simulink model "mpc_test_dist_rej"  (R2024b)
settings: Solver=FixedStepDiscrete  StartTime=0.0  StopTime=10  FixedStep=0.01  RelTol=1e-3  EnableMultiTasking=on
values from neighbouring files (symbols this model uses):
  A_aug = [str_discr_sys.A,str_discr_sys.B ... (first row only)    [MPC_controller.m]    (also in MPC_controller_withint_testing.m)
  B_aug = [str_discr_sys.B;0]    [MPC_controller.m]    (also in MPC_controller_withint_testing.m)
  C_aug = [str_discr_sys.C, zeros(2,1)]    [MPC_controller.m]    (also in MPC_controller_withint_testing.m)
  D_aug = str_discr_sys.D    [MPC_controller.m]    (also in MPC_controller_withint_testing.m)
  h = log(abs(sec(theta)+tan(theta))-C1*alpha)    [Design_of_nonlinear_controller.m]    (also in MPC_controller.m = 0.01; MPC_controller_withint_testing.m = 0.01)
undefined symbols (not defined in the file or in its folder): Discrete, Time
libraries: ctrlSharedLib x1, cstblocks x1
settings Model: Creator=rbabuska  LastModifiedBy=Wesley
settings SolverCC: AlgebraicLoopSolver=TrustRegion
settings DataIOCC: LimitDataPoints=on  SaveFormat=Array  SignalLoggingSaveFormat=ModelDataLogs  ReturnWorkspaceOutputs=off
settings OptimizationCC: ExpressionDepthLimit=2147483647  LifeSpan=inf
settings DebuggingCC: UnderspecifiedInitializationDetection=Classic  MergeDetectMultiDrivingBlocksExec=none  FcnCallInpInsideContextMsg=warning  UnconnectedInputMsg=warning  UnconnectedOutputMsg=warning  UnconnectedLineMsg=warning  StateNameClashWarn=warning  SFUnexpectedBacktrackingDiag=warning  SFNoUnconditionalDefaultTransitionDiag=warning  SFExecutionAtInitializationDiag=none  ArithmeticOperatorsInVariantConditions=warning
settings HardwareCC: ProdBitPerPointer=32  ProdBitPerSizeT=32  ProdBitPerPtrDiffT=32  ProdLargestAtomicFloat=None  ProdIntDivRoundTo=Undefined  ProdEndianess=Unspecified  ProdWordSize=32  ProdHWDeviceType=32-bit Generic
settings ModelReferenceCC: EnableRefExpFcnMdlSchedulingChecks=on  PropagateSignalLabelsOutOfModel=off
settings SFSimCC: SimUseLocalCustomCode=off  CustomCodeUndefinedFunction=UseInterfaceOnly
settings RTWCC: RTWUseLocalCustomCode=off  GPUComputeCapability=3.5  DLArmComputeVersion=19.05
settings CodeAppCC: StateflowObjectComments=on
settings GRTTargetCC: TargetLangStandard=C89/C90 (ANSI)  CombineOutputUpdateFcns=off  GRTInterface=on
settings ConfigComp: CovMetricSettings=dw  CovSaveCumulativeToWorkspaceVar=on  CovSaveSingleToWorkspaceVar=on  CovExternalEMLEnable=off  CovSFcnEnable=off

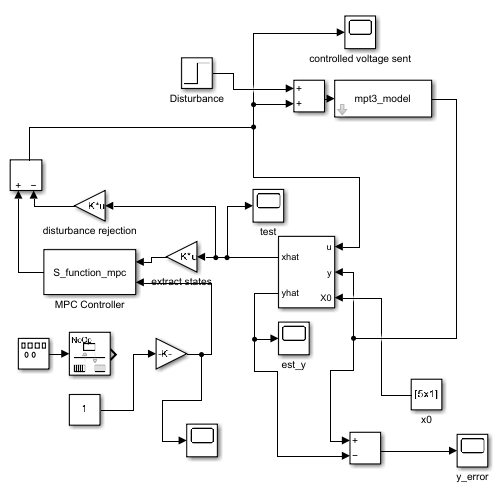
[thumbnail: Simulink's stored preview of the top-level diagram]
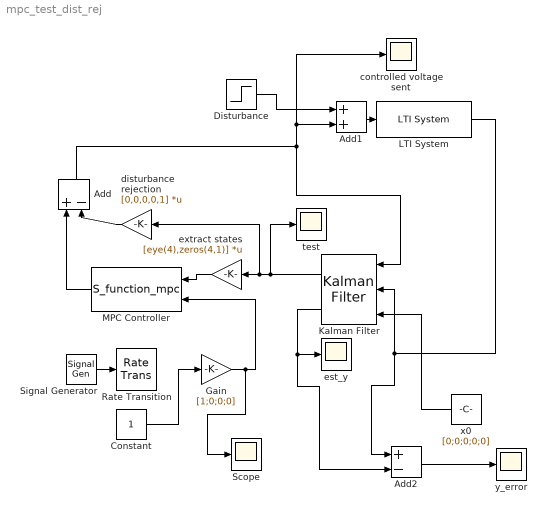
== system mpc_test_dist_rej ==
  Add : Sum  Inputs=+-
  Add1 : Sum
  Add2 : Sum  Inputs=+-
  Constant : Constant
  Disturbance : Step  Time=3  After=0.05  SampleTime=0
  Gain : Gain  Gain=[1;0;0;0]
  Kalman Filter : ctrlSharedLib/Kalman Filter  TimeDomain=Discrete-Time  UseCurrentEstimator=on  ModelSource=Individual A, B, C, D matrices  ModelSourceVariable=ss(0.95,1,1,0,1)  A=A_aug  B=B_aug  C=C_aug  D=D_aug  NumberOfStates=1  NumberOfInputs=1  NumberOfOutputs=1  InitialEstimateSource=Input port  X0=0  P0=10  UseK=off  UseGH=off  NumberOfProcessNoiseInputs=1  G=1  TimeInvariantG=on  H=0  TimeInvariantH=on  Q=blkdiag((1e-2)*eye(4),1e-7)  TimeInvariantQ=on  R=1e-12  TimeInvariantR=on  N=0  TimeInvariantN=on  AddInputPort=on  AddEnablePort=off  OutputEstimatedY=on  OutputP=off  Ts=h
  LTI System : cstblocks/LTI System  sys=mpt3_model  IC=x0  PadeOrder=0
  MPC Controller : M-S-Function  FunctionName=S_function_mpc  Parameters=fast_opt
  Rate Transition : RateTransition  OutPortSampleTime=h
  Scope : Scope
  Signal Generator : SignalGenerator  WaveForm=square  Amplitude=0.5  Frequency=0.11
  controlled voltage sent : Scope
  disturbance rejection : Gain  Gain=[0,0,0,0,1]  Multiplication=Matrix(K*u)
  est_y : Scope
  extract states : Gain  Gain=[eye(4),zeros(4,1)]  Multiplication=Matrix(K*u)
  test : Scope
  x0 : Constant  Value=[0;0;0;0;0]
  y_error : Scope
  wires:
  LTI System/1 -> Add2/1, Kalman Filter/2
  Kalman Filter/2 -> Add2/2, est_y/1
  Add/1 -> controlled voltage sent/1, Add1/2, Kalman Filter/1
  x0/1 -> Kalman Filter/3
  Add2/1 -> y_error/1
  Kalman Filter/1 -> disturbance rejection/1, extract states/1, test/1
  Constant/1 -> Gain/1
  Gain/1 -> Scope/1, MPC Controller/2
  Signal Generator/1 -> Rate Transition/1
  extract states/1 -> MPC Controller/1
  disturbance rejection/1 -> Add/2
  MPC Controller/1 -> Add/1
  Add1/1 -> LTI System/1
  Disturbance/1 -> Add1/1
